simulink model "arm_sim_pid"  (Simulink 7.7)
settings: Solver=ode45  StartTime=0.0  StopTime=100  RelTol=1e-3
undefined symbols (not defined in the file or in its folder): arm_ctrl_pid, drawArm, P
settings Model: Creator=beard  LastModifiedBy=beard
settings OptimizationCC: InitFltsAndDblsToZero=on
settings DebuggingCC: StrictBusMsg=Warning

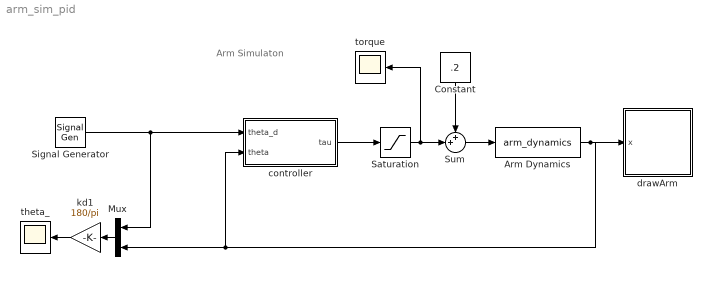
== system arm_sim_pid ==
  note: Arm Simulaton
  Arm Dynamics : S-Function  FunctionName=arm_dynamics  Parameters=AP  EnableBusSupport=off
  Constant : Constant  Value=.2
  Mux : Mux  Inputs=2
  Saturation : Saturate  UpperLimit=P.tau_max  LowerLimit=-P.tau_max
  Signal Generator : SignalGenerator  WaveForm=square  Amplitude=25*pi/180  Frequency=.05
  Sum : Sum  Inputs=++|
  controller : Subsystem
  drawArm : Subsystem
      mask init:
      | % drawing parameters
      | L = 1;
      | w = 0.3;
      mask Display: image(imread('tv.jpg'))
  kd1 : Gain  Gain=180/pi
  theta_ : Scope
      settings: YMin=-30  YMax=35
  torque : Scope
      settings: YMin=0.25  YMax=1.1
  wires:
  Arm Dynamics/1 -> drawArm/1(x), Mux/2, controller/2(theta)
  Mux/1 -> kd1/1
  kd1/1 -> theta_/1
  controller/1(tau) -> Saturation/1
  Signal Generator/1 -> Mux/1, controller/1(theta_d)
  Saturation/1 -> Sum/2, torque/1
  Sum/1 -> Arm Dynamics/1
  Constant/1 -> Sum/1

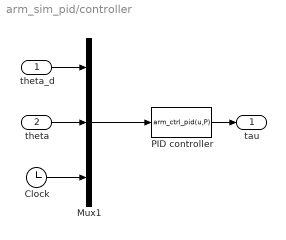
== system arm_sim_pid/controller ==
  theta_d : Inport
  theta : Inport  Port=2
  Clock : Clock
      settings: Decimation=10
  Mux1 : Mux  Inputs=3
  PID controller : MATLABFcn  MATLABFcn=arm_ctrl_pid(u,P)  OutputDimensions=1  SampleTime=P.Ts
  tau : Outport
  wires:
  Mux1/1 -> PID controller/1
  theta_d/1 -> Mux1/1
  theta/1 -> Mux1/2
  PID controller/1 -> tau/1
  Clock/1 -> Mux1/3

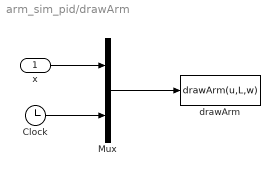
== system arm_sim_pid/drawArm ==
  x : Inport
  Clock : Clock
      settings: Decimation=10
  Mux : Mux  Inputs=2
  drawArm : MATLABFcn  MATLABFcn=drawArm(u,L,w)  OutputDimensions=0  SampleTime=0.1
  wires:
  Mux/1 -> drawArm/1
  x/1 -> Mux/1
  Clock/1 -> Mux/2
